simulink model "task1"  (R2022b)
settings: Solver=FixedStepAuto  StartTime=0.0  StopTime=7  RelTol=1e-8
undefined symbols (not defined in the file): a0, a1, y0, y1
settings Model: Creator=anton  LastModifiedBy=anton
settings DataIOCC: ExternalInput=data  LoadExternalInput=on

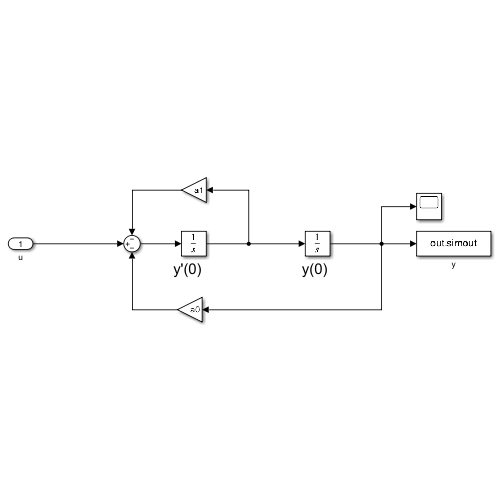
[thumbnail: Simulink's stored preview of the top-level diagram]
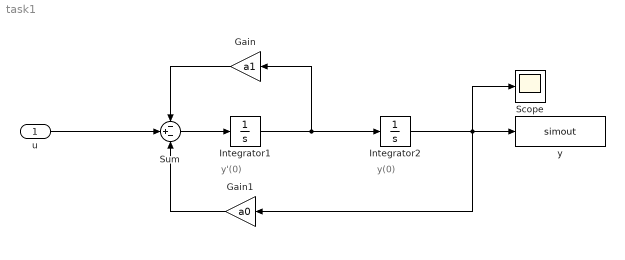
== system task1 ==
  note: y'(0)
  note: y(0)
  u : Inport
  Gain : Gain  Gain=a1
  Gain1 : Gain  Gain=a0
  Integrator1 : Integrator  InitialCondition=y1
  Integrator2 : Integrator  InitialCondition=y0
  Scope : Scope
  Sum : Sum  Inputs=-+-
  y : ToWorkspace  VariableName=simout  SaveFormat=Timeseries  SampleTime=-1
  wires:
  Integrator2/1 -> Scope/1, y/1, Gain1/1
  Integrator1/1 -> Gain/1, Integrator2/1
  u/1 -> Sum/2
  Sum/1 -> Integrator1/1
  Gain/1 -> Sum/1
  Gain1/1 -> Sum/3
